simulink model "TF1_Circuit"  (R2023b)
settings: Solver=VariableStepAuto  StartTime=0.0  StopTime=1.5  RelTol=1e-3
libraries: spsSeriesRLCBranchLib x5, spsGroundLib x4, spsControlledVoltageSourceLib x2, spsVoltageMeasurementLib x2, simulink x1, sps_lib x1
settings Model: Creator=Lucas  LastModifiedBy=Lucas
settings DebuggingCC: AlgebraicLoopMsg=none

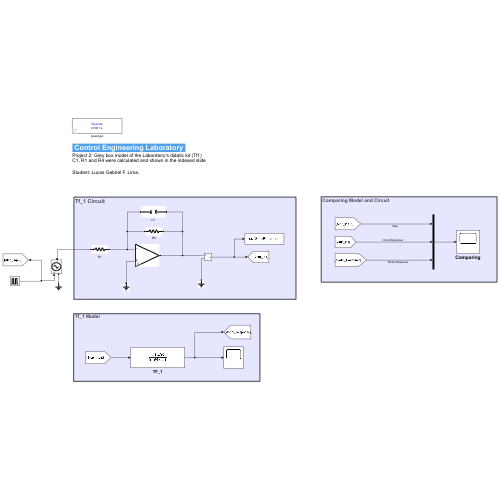
[thumbnail: Simulink's stored preview of the top-level diagram]
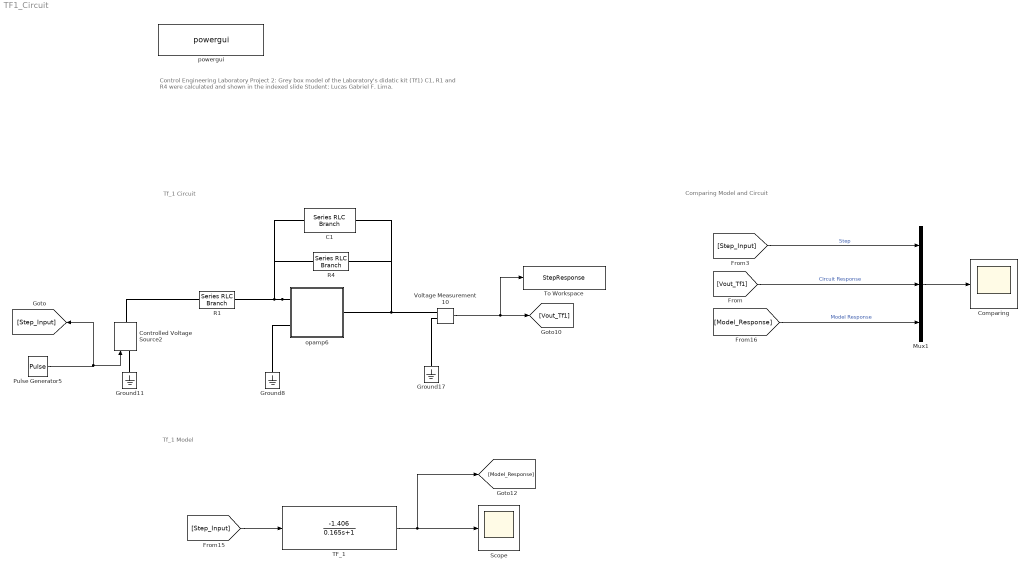
== system TF1_Circuit ==
  note: Tf_1 Circuit
  note: Control Engineering Laboratory
      | Project 2: Grey box model of the Laboratory's didatic kit (Tf1)
      | C1, R1 and R4 were calculated and shown in the indexed slide
      |
      | Student: Lucas Gabriel F. Lima.
  note: Comparing Model and Circuit
  note: Tf_1 Model
  C1 : spsSeriesRLCBranchLib/Series RLC Branch  LConnTagsString=__new0  RConnTagsString=__new0  BranchType=C  Resistance=1  Inductance=1e-3  SetiL0=off  InitialCurrent=0  Capacitance=3.3e-07  Setx0=off  InitialVoltage=0  Measurements=None
  Comparing : Scope
  Controlled Voltage Source2 : spsControlledVoltageSourceLib/Controlled Voltage Source  Initialize=on  Source_Type=AC  Amplitude=0  Phase=0  Frequency=0  Measurements=None
  Ground11 : spsGroundLib/Ground  LConnTagsString=a
  Ground17 : spsGroundLib/Ground  LConnTagsString=a
  Ground8 : spsGroundLib/Ground  LConnTagsString=a
  Mux1 : Mux  Inputs=3
  Pulse Generator5 : DiscretePulseGenerator  PulseType=Time based  Period=3  PulseWidth=50
  R1 : spsSeriesRLCBranchLib/Series RLC Branch  LConnTagsString=__new0  RConnTagsString=__new0  BranchType=R  Resistance=355.62e3  Inductance=1e-3  SetiL0=off  InitialCurrent=0  Capacitance=1e-6  Setx0=off  InitialVoltage=0  Measurements=None
  R4 : spsSeriesRLCBranchLib/Series RLC Branch  LConnTagsString=__new0  RConnTagsString=__new0  BranchType=R  Resistance=500e3  Inductance=1e-3  SetiL0=off  InitialCurrent=0  Capacitance=1e-6  Setx0=off  InitialVoltage=0  Measurements=None
  Scope : Scope
  TF_1 : TransferFcn  Numerator=-1.406  Denominator=[0.165 1]
  To Workspace : ToWorkspace  VariableName=StepResponse  SaveFormat=Structure With Time  SampleTime=-1
  Voltage Measurement10 : spsVoltageMeasurementLib/Voltage Measurement  PhasorSimulation=off  OutputType=Complex  PSBequivalent=0
  opamp6 : Subsystem  mask(Opamp){Ri=1e7, Ro=100, A=200000, U1=12, U2=-12}
      mask prompts: Ri "Input Resistance"; Ro "Output Resistance"; A "Open loop amplification"; U1 "Upper limit supply voltage"; U2 "Lower limit supply voltage"
      mask Display:
      | plot([10 20 30 40], [10 12 14 16],[10 20 30 40], [22 20 18 16],[10 10],[10 22])
      | text(10,13.4,'+')
      | text(10,21,'_')
  powergui : sps_lib/powergui  Priority=1  SimulationMode=Discrete  SampleTime=1e-4  frequency=60  Iterations=50  frequencyindice=0  Pbase=100e6  ErrMax=1e-4  UnitsV=kV  UnitsW=MW  buscounter=0  FunctionMessages=off  echomessages=off  EnableUseOfTLC=off  CurrentSourceSwitches=off  DisableSnubberDevices=off  DisableRonSwitches=off  DisableVfSwitches=off  DisplayEquations=off  AutomaticDiscreteSolvers=off  SolverType=Tustin/Backward Euler (TBE)  Interpol=off  ExternalGateDelay=off  methode=off  Ts=100  x0status=blocks  SPID=off  SwTol=0  HookPort=off  NonlinearTolerance=1e-4  nMaxIteration=100  ContinueOnMaxIteration=off  RestoreLinks=warning  ResistiveCurrentMeasurement=off  Frange=[0:2:500]  Ylog=off  Xlog=on  ShowGrid=off  save=off  variable=ZData  structure=0  ZoomFFT=off  StartTime=0.0  cycles=1  DisplayStyle=1  fundamental=60  FreqAxis=off  MaxFrequency=1000  frequencyindicesteady=1  RmsSteady=1  display=off
  wires:
  Voltage Measurement10/1 -> To Workspace/1, [Vout_Tf1]
  Pulse Generator5/1 -> [Step_Input], Controlled Voltage Source2/1
  [Model_Response] -> Mux1/3  "Model Response"
  [Vout_Tf1] -> Mux1/2  "Circuit Response"
  TF_1/1 -> [Model_Response], Scope/1
  [Step_Input] -> TF_1/1
  [Step_Input] -> Mux1/1  "Step"
  Mux1/1 -> Comparing/1
  connections:
  R1/LConn1 -- Controlled Voltage Source2/RConn1
  opamp6/LConn1 -- C1/LConn1 -- R4/LConn1 -- R1/RConn1
  Controlled Voltage Source2/LConn1 -- Ground11/LConn1
  opamp6/RConn1 -- Voltage Measurement10/LConn1 -- C1/RConn1 -- R4/RConn1
  Ground8/LConn1 -- opamp6/LConn2
  Ground17/LConn1 -- Voltage Measurement10/LConn2

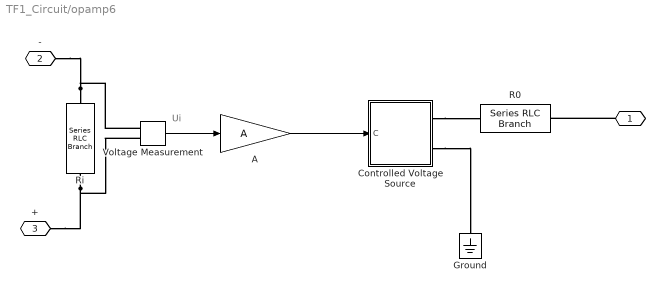
== system TF1_Circuit/opamp6 ==
  note: Ui
  A : Gain  Gain=A
  Controlled Voltage Source : Subsystem
  Ground : spsGroundLib/Ground  LConnTagsString=a
  R0 : spsSeriesRLCBranchLib/Series RLC Branch  LConnTagsString=__new0  RConnTagsString=__new0  BranchType=R  Resistance=Ro  Inductance=1.0  SetiL0=off  InitialCurrent=0  Capacitance=1.0  Setx0=off  InitialVoltage=0  Measurements=None
  Ri : spsSeriesRLCBranchLib/Series RLC Branch  LConnTagsString=__new0  RConnTagsString=__new0  BranchType=R  Resistance=Ri  Inductance=1.0  SetiL0=off  InitialCurrent=0  Capacitance=1.0  Setx0=off  InitialVoltage=0  Measurements=None
  Voltage Measurement : spsVoltageMeasurementLib/Voltage Measurement  PhasorSimulation=off  OutputType=Complex  PSBequivalent=0
  " " : PMIOPort  Side=Right
  - : PMIOPort  Port=2  Side=Left
  + : PMIOPort  Port=3  Side=Left
  wires:
  A/1 -> Controlled Voltage Source/1(C)
  Voltage Measurement/1 -> A/1
  connections:
  Controlled Voltage Source/RConn2 -- Ground/LConn1
  Ri/RConn1 -- Voltage Measurement/LConn2 -- +/RConn1
  Ri/LConn1 -- Voltage Measurement/LConn1 -- -/RConn1
  Controlled Voltage Source/RConn1 -- R0/RConn1
  " "/RConn1 -- R0/LConn1

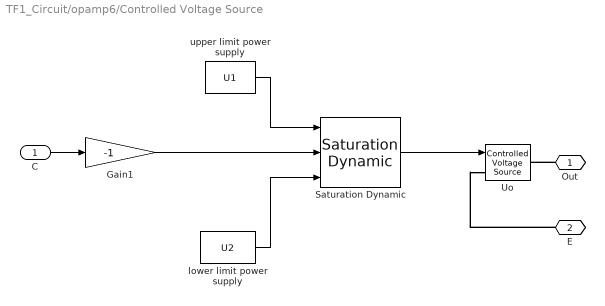
== system TF1_Circuit/opamp6/Controlled Voltage Source ==
  C : Inport
  Gain1 : Gain  Gain=-1
  Saturation Dynamic : simulink/Discontinuities/Saturation Dynamic  OutMin=[]  OutMax=[]  OutDataTypeStr=Inherit: Same as second input  OutDataType=fixdt(1, 16)  OutScaling=2^-10  DoSatur=off
  Uo : spsControlledVoltageSourceLib/Controlled Voltage Source  Initialize=off  Source_Type=AC  Amplitude=0  Phase=0  Frequency=0  Measurements=None
  lower limit power supply : Constant  Value=U2
  upper limit power supply : Constant  Value=U1
  Out : PMIOPort  Side=Right
  E : PMIOPort  Port=2  Side=Right
  wires:
  Gain1/1 -> Saturation Dynamic/2
  lower limit power supply/1 -> Saturation Dynamic/3
  upper limit power supply/1 -> Saturation Dynamic/1
  C/1 -> Gain1/1
  Saturation Dynamic/1 -> Uo/1
  connections:
  Out/RConn1 -- Uo/RConn1
  E/RConn1 -- Uo/LConn1
